simulink model "CTRL_SPECCTRL_FF_BRK_test"  (R2024b)
settings: Solver=VariableStepAuto  StartTime=0.0  StopTime=10.0  RelTol=1e-3
libraries: CTRL_SPECCTRL_FF_BRK x1
settings Model: Creator=blatak  LastModifiedBy=blatak

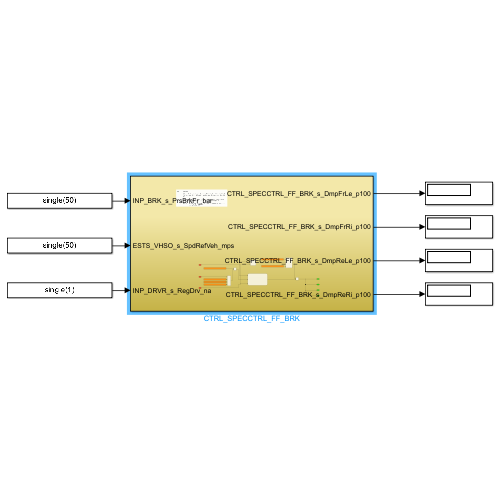
[thumbnail: Simulink's stored preview of the top-level diagram]
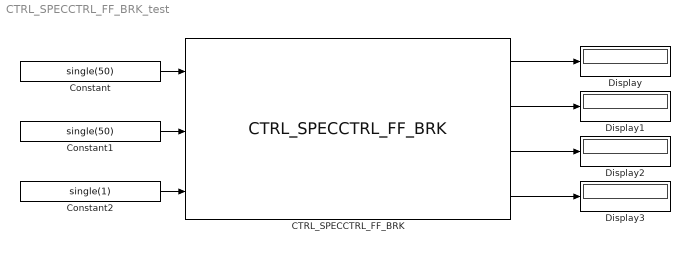
== system CTRL_SPECCTRL_FF_BRK_test ==
  CTRL_SPECCTRL_FF_BRK : CTRL_SPECCTRL_FF_BRK/CTRL_SPECCTRL_FF_BRK  SystemSampleTime=-1  VariantActivationTime=update diagram  AllowFlexibleInterface=on  Latency=0  AutoFrameSizeCalculation=off
  Constant : Constant  Value=single(50)
  Constant1 : Constant  Value=single(50)
  Constant2 : Constant  Value=single(1)
  Display{,1..3} (4 alike) : Display
  wires:
  CTRL_SPECCTRL_FF_BRK/1 -> Display/1
  CTRL_SPECCTRL_FF_BRK/2 -> Display1/1
  CTRL_SPECCTRL_FF_BRK/3 -> Display2/1
  CTRL_SPECCTRL_FF_BRK/4 -> Display3/1
  Constant/1 -> CTRL_SPECCTRL_FF_BRK/1
  Constant1/1 -> CTRL_SPECCTRL_FF_BRK/2
  Constant2/1 -> CTRL_SPECCTRL_FF_BRK/3
